simulink model "stm32f0_can_serial_bridge_binary"  (Simulink 7.3)
settings: Solver=FixedStepDiscrete  SolverMode=SingleTasking  StartTime=0.0  StopTime=10.0  RelTol=1e-3
PreLoadFcn:
  | waijung.modelPreload; % Required for working with Waijung Blockset. Do not remove.
undefined symbols (not defined in the file): LQFP48, STM32F072CB
libraries: simulink x22, stm32f0_can_lib x5, stm32f0_device_config_lib x1
(part 2 of 2)

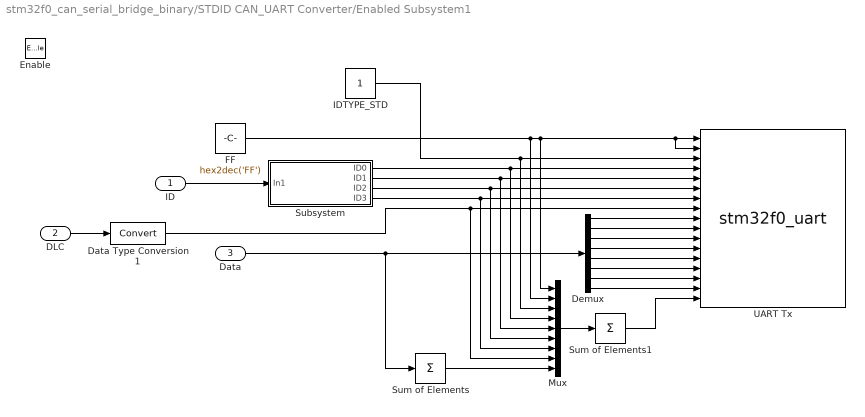
== system stm32f0_can_serial_bridge_binary/STDID CAN_UART Converter/Enabled Subsystem1 ==
  ID : Inport  OutDataType=fixdt(1, 16)  OutScaling=2^0
  DLC : Inport  Port=2  OutDataType=fixdt(1, 16)  OutScaling=2^0
  Data : Inport  Port=3  OutDataType=fixdt(1, 16)  OutScaling=2^0
  Enable : EnablePort
  Data Type Conversion1 : DataTypeConversion  OutDataType=fixdt(1, 16)  OutScaling=2^0
  Demux : Demux  Outputs=8
  FF : Constant  Value=hex2dec('FF')  OutDataTypeMode=uint8  OutDataType=fixdt(1, 16)  OutScaling=2^0  OutDataTypeStr=uint8
  IDTYPE_STD : Constant  OutDataTypeMode=uint8  OutDataType=fixdt(1, 16)  OutScaling=2^0  OutDataTypeStr=uint8
  Mux : Mux  Inputs=9
  Subsystem : Subsystem
  Sum of Elements : Sum  Inputs=+  OutDataType=fixdt(1, 16)  OutScaling=2^-10
  Sum of Elements1 : Sum  Inputs=+  OutDataType=fixdt(1, 16)  OutScaling=2^-10
  UART Tx : S-Function  FunctionName=stm32f0_uart  Parameters=conf,inputporttype,inputportwidth,outputporttype,outputportwidth,asciiheader,optionstring,headerstring,terminatorstring,asciidatatypestring,sampletime,blockid  EnableBusSupport=off  mask(stm32f0_uart){conf=Tx, uartmodule=1, baudrate=115200, databits=8, parity=No, stopbit=1, remaptxpin=A9, remaprxpin=A10, flowcontrol=None, remapctspin=Not used, remaprtspin=Not used, advanceoptions=off, rxbuffersize=64, txbuffersize=64, transfer=Blocking, packetmode=Binary, binheader='', binterminator='', porttype_double=0, porttype_single=0, porttype_int8=0, porttype_uint8=17, porttype_int16=0, porttype_uint16=0, porttype_int32=0, porttype_uint32=0, asciiformat='%u,canrx,extid=%u,dlc=%u,data=%x,%x,%x,%x,%x,%x,%x,%x', rx_asciiterminator=CR (0x0D - "\r"), tx_asciiterminator=CRLF (0x0D 0x0A - "\r\n"), storagename=<empty>, varname=, asciiheader=, sampletime=inf, enablecustomportlabel=off, cinputportlabel=de, coutputportlabel=fff,ff,sdfsd, portpinstr=0, blockid=STDIDCAN_UARTConverterEnabledSubsystem1UARTTx, inputporttype=[3 3 3 3 3 3 3 3 3 3 3 3 3 3 3 3 3], inputportwidth=[], inputportlabel={'uint8' 'uint8' 'uint8' 'uint8' 'uint8' 'uint8' 'uint8' 'uint8' 'uint8' 'uint8' 'uint8' 'uint8' 'uint8' 'uint8' 'uint8' 'uint8' 'uint8'}, outputporttype=[], outputportwidth=[], outputportlabel={}, compat=0, optionstring=["1", "1", "A", "9", "1", "A", "10", "0", "*", "*", "0", "*", "*", "1", "1", "", "", "115200", "8", "No", "1", "None", "3", "2", "64", "64", "Binary", "Blocking", ""], headerstring=[], terminatorstring=[], asciidatatypestring=[], lastmodule=1}
      mask prompts: conf "Configuration"; uartmodule "UART Module"; baudrate "Baud rate (bps)"; databits "Data bits"; stopbit "Stop bit"; remaptxpin "Tx pin"; remaprxpin "Rx pin"; flowcontrol "Hardware flow control"; remapctspin "HW Flow control, CTS Pin"; remaprtspin "HW Flow control, RTS Pin"; advanceoptions "Advance options"; rxbuffersize "Rx buffer size (bytes)"; txbuffersize "Tx buffer size (bytes)"; packetmode "Packet mode"; binheader "Binary header (example: '7E 7E')"; binterminator "Binary terminator (example: '03 03')"; porttype_double "Number of data port, type DOUBLE"; porttype_single "Number of data port, type SINGLE"; porttype_int8 "Number of data port, type INT8"; porttype_uint8 "Number of data port, type UINT8"; porttype_int16 "Number of data port, type INT16"; porttype_uint16 "Number of data port, type UINT16"; porttype_int32 "Number of data port, type INT32"; porttype_uint32 "Number of data port, type UINT32"; asciiformat "Ascii format"; rx_asciiterminator "End of packet"; tx_asciiterminator "End of packet"; storagename "Buffer"; varname "Var name"; asciiheader "Ascii header (printf format)"; sampletime "Sample time (sec)"; enablecustomportlabel "Enable custom port labels (Ex. In1, In2, In3)"; cinputportlabel "Custom input port labels (Ex. In1, In2, In3)"; coutputportlabel "Custom output port labels (Ex. Out1, Out2, Out3)"; portpinstr "Port Pin String"; blockid "Block ID"; inputporttype "Input Port Type"; inputportwidth "Input Port Width"; inputportlabel "Input Port Label"; outputporttype "Output Port Type"; outputportwidth "Output Port Width"; outputportlabel "Output port label"; compat "Compatibility (Reserved for future use)"; optionstring "String(s) to be passed to TLC"; lastmodule "Last module selected"
      mask help:
      | UART Module
      |  - Select module corresponding to "UART Setup" block.
      | Transfer
      |  - Blocking: after write DMA buffer, the block wait until buffer empty.
      |  - Non-Blocking: the block will not wait for buffer empty.
      | Packet mode:
      |  - Ascii: sending data is ascii, Ascii format + End of packet.
      |  - Binary: sending data is binary format, Header + Data + Terminator
      |  - String Buffer: Volatile Data Storage variable name as sending data.
      | Ascii format:
      |  - %U, %I, %D, %O, %X, %u, %i, %d, %o, %x: Uint32
      |  - %E, %G, %F, %e, %g, %f: Single
      |  - %C, %c: Int8
      |  - %S, %s: (char *), this port is output of Volatile Data Storage Read block, which data type is string.
      mask init:
      | stm32f0_uart_callback('init');
      mask Help: web(fullfile(waijungdocroot,'stm32f0_uart_tx.htm'), '-browser')
      mask StyleString: popup(Setup|Tx|Rx),popup(1|2|3|4),edit,popup(8),popup(No|Odd|Even),popup(0.5|1|1.5|2),popup(Not used|A9|B6),popup(Not used|A10|B7),popup(None|RTS|CTS|RTS/CTS),popup(Not used|A11),popup(Not used|A12),checkbox,popup(16|32|64|128|256|512),popup(16|32|64|128|256|512),popup(Blocking|Non-Blocking),popup(Ascii|Binary|String Buffer),edit,edit,edit,edit,edit,edit,edit,edit,edit,edit,edit,popup(CR (0x0D - "\r")|LF (0x0A - "\n")|CRLF (0x0D 0x0A - "\r\n")),popup(CR (0x0D - "\r")|LF (0x0A - "\n")|CRLF (0x0D 0x0A - "\r\n")|None),popup(<empty>),edit,edit,edit,checkbox,edit,edit,edit,edit,edit,edit,edit,edit,edit,edit,edit,edit,edit,edit,edit,edit
      mask CallbackString: stm32f0_uart_callback('conf');|stm32f0_uart_callback('uartmodule');|||||||stm32f0_uart_callback('flowcontrol');|||stm32f0_uart_callback('advanceoptions');|||stm32f0_uart_callback('conf');|stm32f0_uart_callback('conf');|stm32f0_uart_callback('binheader');|stm32f0_uart_callback('binterminator');|||||||||stm32f0_uart_callback('asciiformat');|||stm32f0_uart_callback('storagename');|||stm32f0_uart_callback('sampletime');|stm32f0_uart_callback('enablecustomportlabel');|stm32f0_uart_callback('conf');|stm32f0_uart_callback('conf');||stm32f0_uart_callback('blockid');||||||||||||
      mask Display: text(0.95, 0.5, 'Module: USART1_Tx\nPacket: Binary\nTransfer: Blocking\nTs (sec): 0.001','ver','middle','hor','right'); port_label('input', 1,'uint8'); port_label('input', 2,'uint8'); port_label('input', 3,'uint8'); port_label('input', 4,'uint8'); port_label('input', 5,'uint8'); port_label('input', 6,'uint8'); port_label('input', 7,'uint8'); port_label('input', 8,'uint8'); port_label('input', 9,'uint8'); port_label('input', 10,'uint8'); port_label('input', 11,'uint8'); port_label('input', 12,'uint8'); port_label('input', 13,'uint8'); port_label('input', 14,'uint8'); port_label('input', 15,'uint8'); port_label('input', 16,'uint8'); port_label('input', 17,'uint8');
  wires:
  DLC/1 -> Data Type Conversion1/1
  FF/1 -> UART Tx/1, UART Tx/2, Mux/1, Mux/2
  IDTYPE_STD/1 -> UART Tx/3, Mux/3
  Subsystem/1(ID0) -> UART Tx/4, Mux/4
  Subsystem/2(ID1) -> UART Tx/5, Mux/5
  Subsystem/3(ID2) -> UART Tx/6, Mux/6
  Subsystem/4(ID3) -> UART Tx/7, Mux/7
  ID/1 -> Subsystem/1(In1)
  Data Type Conversion1/1 -> UART Tx/8, Mux/8
  Demux/1 -> UART Tx/9
  Demux/2 -> UART Tx/10
  Demux/3 -> UART Tx/11
  Demux/4 -> UART Tx/12
  Demux/5 -> UART Tx/13
  Demux/6 -> UART Tx/14
  Demux/7 -> UART Tx/15
  Demux/8 -> UART Tx/16
  Data/1 -> Demux/1, Sum of Elements/1
  Sum of Elements/1 -> Mux/9
  Mux/1 -> Sum of Elements1/1
  Sum of Elements1/1 -> UART Tx/17

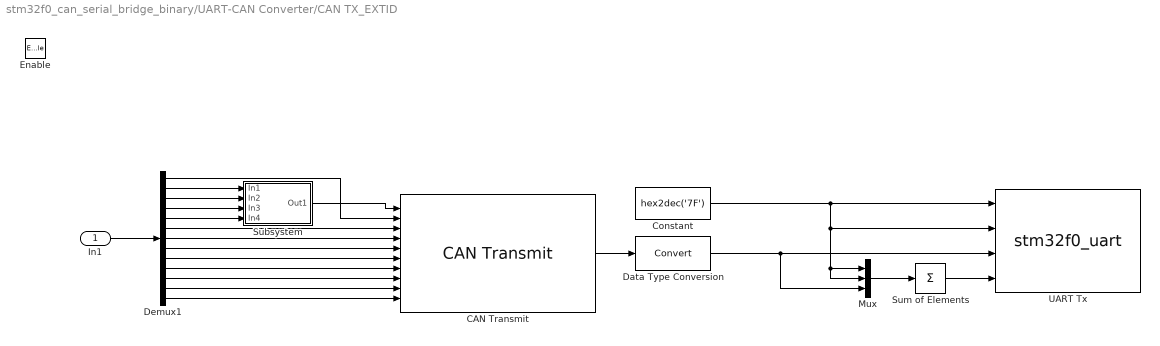
== system stm32f0_can_serial_bridge_binary/UART-CAN Converter/CAN TX_EXTID ==
  In1 : Inport  OutDataType=fixdt(1, 16)  OutScaling=2^0
  Enable : EnablePort
  CAN Transmit : stm32f0_can_lib/CAN Transmit  conf=Tx  canmodule=1  transfer=Blocking  timeout=0.5  idtype=Extended  specificid=off  id=0  specificdlc=off  dlc=8  enablestatus=on  datatype=single  data0type=uint8  data1type=uint8  data2type=uint8  data3type=uint8  data4type=uint8  data5type=uint8  data6type=uint8  data7type=uint8  inputarray=[ -1, -1, 3, 3, 3, 3, 3, 3, 3, 3]  inputlabelarray={ 'ID', 'DLC', 'D0 (uint8)', 'D1 (uint8)', 'D2 (uint8)', 'D3 (uint8)', 'D4 (uint8)', 'D5 (uint8)', 'D6 (uint8)', 'D7 (uint8)' }  outputarray=[7]  outputlabelarray={'Status'}  sampletime=-1  sampletimestr=0.001  blockid=UARTCANConverterCANTX_EXTIDCANTransmit  compat=0  confstr="[\"Blocking\",\"0.5\",\"Extended\",\"off\",\"0\",\"off\",\"8\",\"on\",\"uint8\",\"uint8\",\"uint8\",\"uint8\",\"uint8\",\"uint8\",\"uint8\",\"uint8\"]"
  Constant : Constant  Value=hex2dec('7F')  OutDataTypeMode=uint8  OutDataType=fixdt(1, 16)  OutScaling=2^0  OutDataTypeStr=uint8
  Data Type Conversion : DataTypeConversion  OutDataType=fixdt(1, 16)  OutScaling=2^0
  Demux1 : Demux  Outputs=13
  Mux : Mux  Inputs=3
  Subsystem : Subsystem
  Sum of Elements : Sum  Inputs=+  OutDataType=fixdt(1, 16)  OutScaling=2^-10
  UART Tx : S-Function  FunctionName=stm32f0_uart  Parameters=conf,inputporttype,inputportwidth,outputporttype,outputportwidth,asciiheader,optionstring,headerstring,terminatorstring,asciidatatypestring,sampletime,blockid  EnableBusSupport=off  mask(stm32f0_uart){conf=Tx, uartmodule=1, baudrate=115200, databits=8, parity=No, stopbit=1, remaptxpin=A9, remaprxpin=A10, flowcontrol=None, remapctspin=Not used, remaprtspin=Not used, advanceoptions=off, rxbuffersize=64, txbuffersize=64, transfer=Blocking, packetmode=Binary, binheader='', binterminator='', porttype_double=0, porttype_single=0, porttype_int8=0, porttype_uint8=4, porttype_int16=0, porttype_uint16=0, porttype_int32=0, porttype_uint32=0, asciiformat='%u: CODE: %u', rx_asciiterminator=CR (0x0D - "\r"), tx_asciiterminator=CRLF (0x0D 0x0A - "\r\n"), storagename=<empty>, varname=, asciiheader=, sampletime=inf, enablecustomportlabel=off, cinputportlabel=de, coutputportlabel=fff,ff,sdfsd, portpinstr=0, blockid=UARTCANConverterCANTX_EXTIDUARTTx, inputporttype=[3 3 3 3], inputportwidth=[], inputportlabel={'uint8' 'uint8' 'uint8' 'uint8'}, outputporttype=[], outputportwidth=[], outputportlabel={}, compat=0, optionstring=["1", "1", "A", "9", "1", "A", "10", "0", "*", "*", "0", "*", "*", "1", "1", "", "", "115200", "8", "No", "1", "None", "3", "2", "64", "64", "Binary", "Blocking", ""], headerstring=[], terminatorstring=[], asciidatatypestring=[], lastmodule=1}
      mask prompts: conf "Configuration"; uartmodule "UART Module"; baudrate "Baud rate (bps)"; databits "Data bits"; stopbit "Stop bit"; remaptxpin "Tx pin"; remaprxpin "Rx pin"; flowcontrol "Hardware flow control"; remapctspin "HW Flow control, CTS Pin"; remaprtspin "HW Flow control, RTS Pin"; advanceoptions "Advance options"; rxbuffersize "Rx buffer size (bytes)"; txbuffersize "Tx buffer size (bytes)"; packetmode "Packet mode"; binheader "Binary header (example: '7E 7E')"; binterminator "Binary terminator (example: '03 03')"; porttype_double "Number of data port, type DOUBLE"; porttype_single "Number of data port, type SINGLE"; porttype_int8 "Number of data port, type INT8"; porttype_uint8 "Number of data port, type UINT8"; porttype_int16 "Number of data port, type INT16"; porttype_uint16 "Number of data port, type UINT16"; porttype_int32 "Number of data port, type INT32"; porttype_uint32 "Number of data port, type UINT32"; asciiformat "Ascii format"; rx_asciiterminator "End of packet"; tx_asciiterminator "End of packet"; storagename "Buffer"; varname "Var name"; asciiheader "Ascii header (printf format)"; sampletime "Sample time (sec)"; enablecustomportlabel "Enable custom port labels (Ex. In1, In2, In3)"; cinputportlabel "Custom input port labels (Ex. In1, In2, In3)"; coutputportlabel "Custom output port labels (Ex. Out1, Out2, Out3)"; portpinstr "Port Pin String"; blockid "Block ID"; inputporttype "Input Port Type"; inputportwidth "Input Port Width"; inputportlabel "Input Port Label"; outputporttype "Output Port Type"; outputportwidth "Output Port Width"; outputportlabel "Output port label"; compat "Compatibility (Reserved for future use)"; optionstring "String(s) to be passed to TLC"; lastmodule "Last module selected"
      mask help:
      | UART Module
      |  - Select module corresponding to "UART Setup" block.
      | Transfer
      |  - Blocking: after write DMA buffer, the block wait until buffer empty.
      |  - Non-Blocking: the block will not wait for buffer empty.
      | Packet mode:
      |  - Ascii: sending data is ascii, Ascii format + End of packet.
      |  - Binary: sending data is binary format, Header + Data + Terminator
      |  - String Buffer: Volatile Data Storage variable name as sending data.
      | Ascii format:
      |  - %U, %I, %D, %O, %X, %u, %i, %d, %o, %x: Uint32
      |  - %E, %G, %F, %e, %g, %f: Single
      |  - %C, %c: Int8
      |  - %S, %s: (char *), this port is output of Volatile Data Storage Read block, which data type is string.
      mask init:
      | stm32f0_uart_callback('init');
      mask Help: web(fullfile(waijungdocroot,'stm32f0_uart_tx.htm'), '-browser')
      mask StyleString: popup(Setup|Tx|Rx),popup(1|2|3|4),edit,popup(8),popup(No|Odd|Even),popup(0.5|1|1.5|2),popup(Not used|A9|B6),popup(Not used|A10|B7),popup(None|RTS|CTS|RTS/CTS),popup(Not used|A11),popup(Not used|A12),checkbox,popup(16|32|64|128|256|512),popup(16|32|64|128|256|512),popup(Blocking|Non-Blocking),popup(Ascii|Binary|String Buffer),edit,edit,edit,edit,edit,edit,edit,edit,edit,edit,edit,popup(CR (0x0D - "\r")|LF (0x0A - "\n")|CRLF (0x0D 0x0A - "\r\n")),popup(CR (0x0D - "\r")|LF (0x0A - "\n")|CRLF (0x0D 0x0A - "\r\n")|None),popup(<empty>),edit,edit,edit,checkbox,edit,edit,edit,edit,edit,edit,edit,edit,edit,edit,edit,edit,edit,edit,edit,edit
      mask CallbackString: stm32f0_uart_callback('conf');|stm32f0_uart_callback('uartmodule');|||||||stm32f0_uart_callback('flowcontrol');|||stm32f0_uart_callback('advanceoptions');|||stm32f0_uart_callback('conf');|stm32f0_uart_callback('conf');|stm32f0_uart_callback('binheader');|stm32f0_uart_callback('binterminator');|||||||||stm32f0_uart_callback('asciiformat');|||stm32f0_uart_callback('storagename');|||stm32f0_uart_callback('sampletime');|stm32f0_uart_callback('enablecustomportlabel');|stm32f0_uart_callback('conf');|stm32f0_uart_callback('conf');||stm32f0_uart_callback('blockid');||||||||||||
      mask Display: text(0.95, 0.5, 'Module: USART1_Tx\nPacket: Binary\nTransfer: Blocking\nTs (sec): 0.001','ver','middle','hor','right'); port_label('input', 1,'uint8'); port_label('input', 2,'uint8'); port_label('input', 3,'uint8'); port_label('input', 4,'uint8');
  wires:
  CAN Transmit/1 -> Data Type Conversion/1
  Demux1/13 -> CAN Transmit/10
  Demux1/12 -> CAN Transmit/9
  Demux1/11 -> CAN Transmit/8
  Demux1/10 -> CAN Transmit/7
  Demux1/9 -> CAN Transmit/6
  Demux1/8 -> CAN Transmit/5
  Demux1/7 -> CAN Transmit/4
  Demux1/6 -> CAN Transmit/3
  Demux1/1 -> CAN Transmit/2
  In1/1 -> Demux1/1
  Demux1/2 -> Subsystem/1(In1)
  Demux1/3 -> Subsystem/2(In2)
  Demux1/4 -> Subsystem/3(In3)
  Demux1/5 -> Subsystem/4(In4)
  Subsystem/1(Out1) -> CAN Transmit/1
  Mux/1 -> Sum of Elements/1
  Data Type Conversion/1 -> UART Tx/3, Mux/3
  Sum of Elements/1 -> UART Tx/4
  Constant/1 -> UART Tx/1, UART Tx/2, Mux/1, Mux/2

== system stm32f0_can_serial_bridge_binary/UART-CAN Converter/CAN TX_STDID ==
  In1 : Inport  OutDataType=fixdt(1, 16)  OutScaling=2^0
  Enable : EnablePort
  CAN Transmit : stm32f0_can_lib/CAN Transmit  conf=Tx  canmodule=1  transfer=Blocking  timeout=0.5  idtype=Standard  specificid=off  id=0  specificdlc=off  dlc=8  enablestatus=on  datatype=single  data0type=uint8  data1type=uint8  data2type=uint8  data3type=uint8  data4type=uint8  data5type=uint8  data6type=uint8  data7type=uint8  inputarray=[ -1, -1, 3, 3, 3, 3, 3, 3, 3, 3]  inputlabelarray={ 'ID', 'DLC', 'D0 (uint8)', 'D1 (uint8)', 'D2 (uint8)', 'D3 (uint8)', 'D4 (uint8)', 'D5 (uint8)', 'D6 (uint8)', 'D7 (uint8)' }  outputarray=[7]  outputlabelarray={'Status'}  sampletime=-1  sampletimestr=0.001  blockid=UARTCANConverterCANTX_STDIDCANTransmit  compat=0  confstr="[\"Blocking\",\"0.5\",\"Standard\",\"off\",\"0\",\"off\",\"8\",\"on\",\"uint8\",\"uint8\",\"uint8\",\"uint8\",\"uint8\",\"uint8\",\"uint8\",\"uint8\"]"
  Constant : Constant  Value=hex2dec('7F')  OutDataTypeMode=uint8  OutDataType=fixdt(1, 16)  OutScaling=2^0  OutDataTypeStr=uint8
  Data Type Conversion : DataTypeConversion  OutDataType=fixdt(1, 16)  OutScaling=2^0
  Demux2 : Demux  Outputs=13
  Mux : Mux  Inputs=3
  Subsystem : Subsystem
  Sum of Elements : Sum  Inputs=+  OutDataType=fixdt(1, 16)  OutScaling=2^-10
  UART Tx : S-Function  FunctionName=stm32f0_uart  Parameters=conf,inputporttype,inputportwidth,outputporttype,outputportwidth,asciiheader,optionstring,headerstring,terminatorstring,asciidatatypestring,sampletime,blockid  EnableBusSupport=off  mask(stm32f0_uart){conf=Tx, uartmodule=1, baudrate=115200, databits=8, parity=No, stopbit=1, remaptxpin=A9, remaprxpin=A10, flowcontrol=None, remapctspin=Not used, remaprtspin=Not used, advanceoptions=off, rxbuffersize=64, txbuffersize=64, transfer=Blocking, packetmode=Binary, binheader='', binterminator='', porttype_double=0, porttype_single=0, porttype_int8=0, porttype_uint8=4, porttype_int16=0, porttype_uint16=0, porttype_int32=0, porttype_uint32=0, asciiformat='%u: CODE: %u', rx_asciiterminator=CR (0x0D - "\r"), tx_asciiterminator=CRLF (0x0D 0x0A - "\r\n"), storagename=<empty>, varname=, asciiheader=, sampletime=inf, enablecustomportlabel=off, cinputportlabel=de, coutputportlabel=fff,ff,sdfsd, portpinstr=0, blockid=UARTCANConverterCANTX_STDIDUARTTx, inputporttype=[3 3 3 3], inputportwidth=[], inputportlabel={'uint8' 'uint8' 'uint8' 'uint8'}, outputporttype=[], outputportwidth=[], outputportlabel={}, compat=0, optionstring=["1", "1", "A", "9", "1", "A", "10", "0", "*", "*", "0", "*", "*", "1", "1", "", "", "115200", "8", "No", "1", "None", "3", "2", "64", "64", "Binary", "Blocking", ""], headerstring=[], terminatorstring=[], asciidatatypestring=[], lastmodule=1}
      mask prompts: conf "Configuration"; uartmodule "UART Module"; baudrate "Baud rate (bps)"; databits "Data bits"; stopbit "Stop bit"; remaptxpin "Tx pin"; remaprxpin "Rx pin"; flowcontrol "Hardware flow control"; remapctspin "HW Flow control, CTS Pin"; remaprtspin "HW Flow control, RTS Pin"; advanceoptions "Advance options"; rxbuffersize "Rx buffer size (bytes)"; txbuffersize "Tx buffer size (bytes)"; packetmode "Packet mode"; binheader "Binary header (example: '7E 7E')"; binterminator "Binary terminator (example: '03 03')"; porttype_double "Number of data port, type DOUBLE"; porttype_single "Number of data port, type SINGLE"; porttype_int8 "Number of data port, type INT8"; porttype_uint8 "Number of data port, type UINT8"; porttype_int16 "Number of data port, type INT16"; porttype_uint16 "Number of data port, type UINT16"; porttype_int32 "Number of data port, type INT32"; porttype_uint32 "Number of data port, type UINT32"; asciiformat "Ascii format"; rx_asciiterminator "End of packet"; tx_asciiterminator "End of packet"; storagename "Buffer"; varname "Var name"; asciiheader "Ascii header (printf format)"; sampletime "Sample time (sec)"; enablecustomportlabel "Enable custom port labels (Ex. In1, In2, In3)"; cinputportlabel "Custom input port labels (Ex. In1, In2, In3)"; coutputportlabel "Custom output port labels (Ex. Out1, Out2, Out3)"; portpinstr "Port Pin String"; blockid "Block ID"; inputporttype "Input Port Type"; inputportwidth "Input Port Width"; inputportlabel "Input Port Label"; outputporttype "Output Port Type"; outputportwidth "Output Port Width"; outputportlabel "Output port label"; compat "Compatibility (Reserved for future use)"; optionstring "String(s) to be passed to TLC"; lastmodule "Last module selected"
      mask help:
      | UART Module
      |  - Select module corresponding to "UART Setup" block.
      | Transfer
      |  - Blocking: after write DMA buffer, the block wait until buffer empty.
      |  - Non-Blocking: the block will not wait for buffer empty.
      | Packet mode:
      |  - Ascii: sending data is ascii, Ascii format + End of packet.
      |  - Binary: sending data is binary format, Header + Data + Terminator
      |  - String Buffer: Volatile Data Storage variable name as sending data.
      | Ascii format:
      |  - %U, %I, %D, %O, %X, %u, %i, %d, %o, %x: Uint32
      |  - %E, %G, %F, %e, %g, %f: Single
      |  - %C, %c: Int8
      |  - %S, %s: (char *), this port is output of Volatile Data Storage Read block, which data type is string.
      mask init:
      | stm32f0_uart_callback('init');
      mask Help: web(fullfile(waijungdocroot,'stm32f0_uart_tx.htm'), '-browser')
      mask StyleString: popup(Setup|Tx|Rx),popup(1|2|3|4),edit,popup(8),popup(No|Odd|Even),popup(0.5|1|1.5|2),popup(Not used|A9|B6),popup(Not used|A10|B7),popup(None|RTS|CTS|RTS/CTS),popup(Not used|A11),popup(Not used|A12),checkbox,popup(16|32|64|128|256|512),popup(16|32|64|128|256|512),popup(Blocking|Non-Blocking),popup(Ascii|Binary|String Buffer),edit,edit,edit,edit,edit,edit,edit,edit,edit,edit,edit,popup(CR (0x0D - "\r")|LF (0x0A - "\n")|CRLF (0x0D 0x0A - "\r\n")),popup(CR (0x0D - "\r")|LF (0x0A - "\n")|CRLF (0x0D 0x0A - "\r\n")|None),popup(<empty>),edit,edit,edit,checkbox,edit,edit,edit,edit,edit,edit,edit,edit,edit,edit,edit,edit,edit,edit,edit,edit
      mask CallbackString: stm32f0_uart_callback('conf');|stm32f0_uart_callback('uartmodule');|||||||stm32f0_uart_callback('flowcontrol');|||stm32f0_uart_callback('advanceoptions');|||stm32f0_uart_callback('conf');|stm32f0_uart_callback('conf');|stm32f0_uart_callback('binheader');|stm32f0_uart_callback('binterminator');|||||||||stm32f0_uart_callback('asciiformat');|||stm32f0_uart_callback('storagename');|||stm32f0_uart_callback('sampletime');|stm32f0_uart_callback('enablecustomportlabel');|stm32f0_uart_callback('conf');|stm32f0_uart_callback('conf');||stm32f0_uart_callback('blockid');||||||||||||
      mask Display: text(0.95, 0.5, 'Module: USART1_Tx\nPacket: Binary\nTransfer: Blocking\nTs (sec): 0.001','ver','middle','hor','right'); port_label('input', 1,'uint8'); port_label('input', 2,'uint8'); port_label('input', 3,'uint8'); port_label('input', 4,'uint8');
  wires:
  CAN Transmit/1 -> Data Type Conversion/1
  In1/1 -> Demux2/1
  Demux2/13 -> CAN Transmit/10
  Demux2/6 -> CAN Transmit/3
  Demux2/7 -> CAN Transmit/4
  Demux2/8 -> CAN Transmit/5
  Demux2/9 -> CAN Transmit/6
  Demux2/10 -> CAN Transmit/7
  Demux2/11 -> CAN Transmit/8
  Demux2/12 -> CAN Transmit/9
  Demux2/1 -> Subsystem/1(In1)
  Demux2/2 -> Subsystem/2(In2)
  Demux2/3 -> Subsystem/3(In3)
  Demux2/4 -> Subsystem/4(In4)
  Subsystem/1(Out1) -> CAN Transmit/1
  Demux2/5 -> CAN Transmit/2
  Data Type Conversion/1 -> UART Tx/3, Mux/3
  Mux/1 -> Sum of Elements/1
  Constant/1 -> UART Tx/1, Mux/1, Mux/2, UART Tx/2
  Sum of Elements/1 -> UART Tx/4

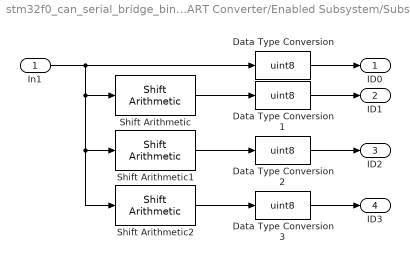
== system stm32f0_can_serial_bridge_binary/EXTID CAN-UART Converter/Enabled Subsystem/Subsystem ==
  In1 : Inport  OutDataType=fixdt(1, 16)  OutScaling=2^0
  Data Type Conversion{,1..3} (4 alike) : DataTypeConversion  OutDataTypeMode=uint8  OutDataType=fixdt(1, 16)  OutScaling=2^0  OutDataTypeStr=uint8
  Shift Arithmetic : simulink/Logic and Bit Operations/Shift Arithmetic  SystemSampleTime=-1  nBitShiftRight=8  nBinPtShiftRight=0
  Shift Arithmetic1 : simulink/Logic and Bit Operations/Shift Arithmetic  SystemSampleTime=-1  nBitShiftRight=16  nBinPtShiftRight=0
  Shift Arithmetic2 : simulink/Logic and Bit Operations/Shift Arithmetic  SystemSampleTime=-1  nBitShiftRight=24  nBinPtShiftRight=0
  ID0 : Outport  OutDataType=fixdt(1, 16)  OutScaling=2^0
  ID1 : Outport  Port=2  OutDataType=fixdt(1, 16)  OutScaling=2^0
  ID2 : Outport  Port=3  OutDataType=fixdt(1, 16)  OutScaling=2^0
  ID3 : Outport  Port=4  OutDataType=fixdt(1, 16)  OutScaling=2^0
  wires:
  In1/1 -> Data Type Conversion/1, Shift Arithmetic/1, Shift Arithmetic1/1, Shift Arithmetic2/1
  Data Type Conversion/1 -> ID0/1
  Shift Arithmetic/1 -> Data Type Conversion1/1
  Shift Arithmetic1/1 -> Data Type Conversion2/1
  Shift Arithmetic2/1 -> Data Type Conversion3/1
  Data Type Conversion1/1 -> ID1/1
  Data Type Conversion2/1 -> ID2/1
  Data Type Conversion3/1 -> ID3/1

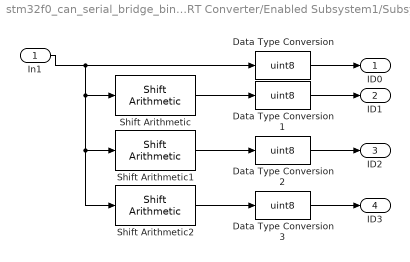
== system stm32f0_can_serial_bridge_binary/STDID CAN_UART Converter/Enabled Subsystem1/Subsystem ==
  In1 : Inport  OutDataType=fixdt(1, 16)  OutScaling=2^0
  Data Type Conversion{,1..3} (4 alike) : DataTypeConversion  OutDataTypeMode=uint8  OutDataType=fixdt(1, 16)  OutScaling=2^0  OutDataTypeStr=uint8
  Shift Arithmetic : simulink/Logic and Bit Operations/Shift Arithmetic  SystemSampleTime=-1  nBitShiftRight=8  nBinPtShiftRight=0
  Shift Arithmetic1 : simulink/Logic and Bit Operations/Shift Arithmetic  SystemSampleTime=-1  nBitShiftRight=16  nBinPtShiftRight=0
  Shift Arithmetic2 : simulink/Logic and Bit Operations/Shift Arithmetic  SystemSampleTime=-1  nBitShiftRight=24  nBinPtShiftRight=0
  ID0 : Outport  OutDataType=fixdt(1, 16)  OutScaling=2^0
  ID1 : Outport  Port=2  OutDataType=fixdt(1, 16)  OutScaling=2^0
  ID2 : Outport  Port=3  OutDataType=fixdt(1, 16)  OutScaling=2^0
  ID3 : Outport  Port=4  OutDataType=fixdt(1, 16)  OutScaling=2^0
  wires:
  In1/1 -> Data Type Conversion/1, Shift Arithmetic/1, Shift Arithmetic1/1, Shift Arithmetic2/1
  Data Type Conversion/1 -> ID0/1
  Shift Arithmetic/1 -> Data Type Conversion1/1
  Shift Arithmetic1/1 -> Data Type Conversion2/1
  Shift Arithmetic2/1 -> Data Type Conversion3/1
  Data Type Conversion1/1 -> ID1/1
  Data Type Conversion2/1 -> ID2/1
  Data Type Conversion3/1 -> ID3/1

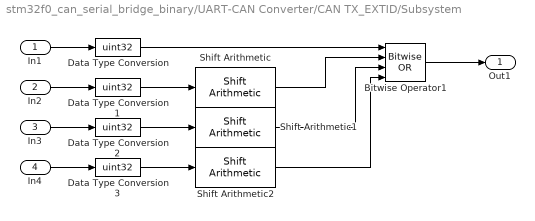
== system stm32f0_can_serial_bridge_binary/UART-CAN Converter/CAN TX_EXTID/Subsystem ==
  In1 : Inport  OutDataType=fixdt(1, 16)  OutScaling=2^0
  In2 : Inport  Port=2  OutDataType=fixdt(1, 16)  OutScaling=2^0
  In3 : Inport  Port=3  OutDataType=fixdt(1, 16)  OutScaling=2^0
  In4 : Inport  Port=4  OutDataType=fixdt(1, 16)  OutScaling=2^0
  Bitwise Operator1 : simulink/Logic and Bit Operations/Bitwise Operator  logicop=OR  UseBitMask=off  NumInputPorts=4  BitMask=bin2dec('11011001')  BitMaskRealWorld=Stored Integer
  Data Type Conversion{,1..3} (4 alike) : DataTypeConversion  OutDataTypeMode=uint32  OutDataType=fixdt(1, 16)  OutScaling=2^0  OutDataTypeStr=uint32
  Shift Arithmetic : simulink/Logic and Bit Operations/Shift Arithmetic  SystemSampleTime=-1  nBitShiftRight=-8  nBinPtShiftRight=0
  Shift Arithmetic1 : simulink/Logic and Bit Operations/Shift Arithmetic  SystemSampleTime=-1  nBitShiftRight=-16  nBinPtShiftRight=0
  Shift Arithmetic2 : simulink/Logic and Bit Operations/Shift Arithmetic  SystemSampleTime=-1  nBitShiftRight=-24  nBinPtShiftRight=0
  Out1 : Outport  OutDataType=fixdt(1, 16)  OutScaling=2^0
  wires:
  In1/1 -> Data Type Conversion/1
  In2/1 -> Data Type Conversion1/1
  In3/1 -> Data Type Conversion2/1
  In4/1 -> Data Type Conversion3/1
  Data Type Conversion1/1 -> Shift Arithmetic/1
  Data Type Conversion2/1 -> Shift Arithmetic1/1
  Data Type Conversion3/1 -> Shift Arithmetic2/1
  Data Type Conversion/1 -> Bitwise Operator1/1
  Shift Arithmetic/1 -> Bitwise Operator1/2
  Shift Arithmetic1/1 -> Bitwise Operator1/3
  Shift Arithmetic2/1 -> Bitwise Operator1/4
  Bitwise Operator1/1 -> Out1/1

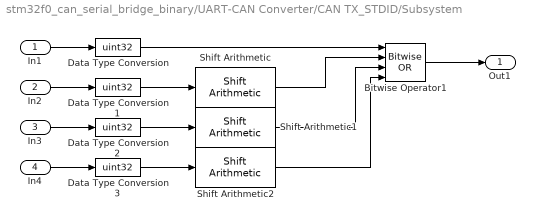
== system stm32f0_can_serial_bridge_binary/UART-CAN Converter/CAN TX_STDID/Subsystem ==
  In1 : Inport  OutDataType=fixdt(1, 16)  OutScaling=2^0
  In2 : Inport  Port=2  OutDataType=fixdt(1, 16)  OutScaling=2^0
  In3 : Inport  Port=3  OutDataType=fixdt(1, 16)  OutScaling=2^0
  In4 : Inport  Port=4  OutDataType=fixdt(1, 16)  OutScaling=2^0
  Bitwise Operator1 : simulink/Logic and Bit Operations/Bitwise Operator  logicop=OR  UseBitMask=off  NumInputPorts=4  BitMask=bin2dec('11011001')  BitMaskRealWorld=Stored Integer
  Data Type Conversion{,1..3} (4 alike) : DataTypeConversion  OutDataTypeMode=uint32  OutDataType=fixdt(1, 16)  OutScaling=2^0  OutDataTypeStr=uint32
  Shift Arithmetic : simulink/Logic and Bit Operations/Shift Arithmetic  SystemSampleTime=-1  nBitShiftRight=-8  nBinPtShiftRight=0
  Shift Arithmetic1 : simulink/Logic and Bit Operations/Shift Arithmetic  SystemSampleTime=-1  nBitShiftRight=-16  nBinPtShiftRight=0
  Shift Arithmetic2 : simulink/Logic and Bit Operations/Shift Arithmetic  SystemSampleTime=-1  nBitShiftRight=-24  nBinPtShiftRight=0
  Out1 : Outport  OutDataType=fixdt(1, 16)  OutScaling=2^0
  wires:
  In1/1 -> Data Type Conversion/1
  In2/1 -> Data Type Conversion1/1
  In3/1 -> Data Type Conversion2/1
  In4/1 -> Data Type Conversion3/1
  Data Type Conversion1/1 -> Shift Arithmetic/1
  Data Type Conversion2/1 -> Shift Arithmetic1/1
  Data Type Conversion3/1 -> Shift Arithmetic2/1
  Data Type Conversion/1 -> Bitwise Operator1/1
  Shift Arithmetic/1 -> Bitwise Operator1/2
  Shift Arithmetic1/1 -> Bitwise Operator1/3
  Shift Arithmetic2/1 -> Bitwise Operator1/4
  Bitwise Operator1/1 -> Out1/1
